simulink model "NEST"  (R2019a)
settings: Solver=VariableStepAuto  StartTime=0.0  StopTime=Inf  RelTol=1e-3
settings Model: Creator=marco  LastModifiedBy=luca
settings DataIOCC: ReturnWorkspaceOutputs=off
settings DebuggingCC: ArithmeticOperatorsInVariantConditions=warning

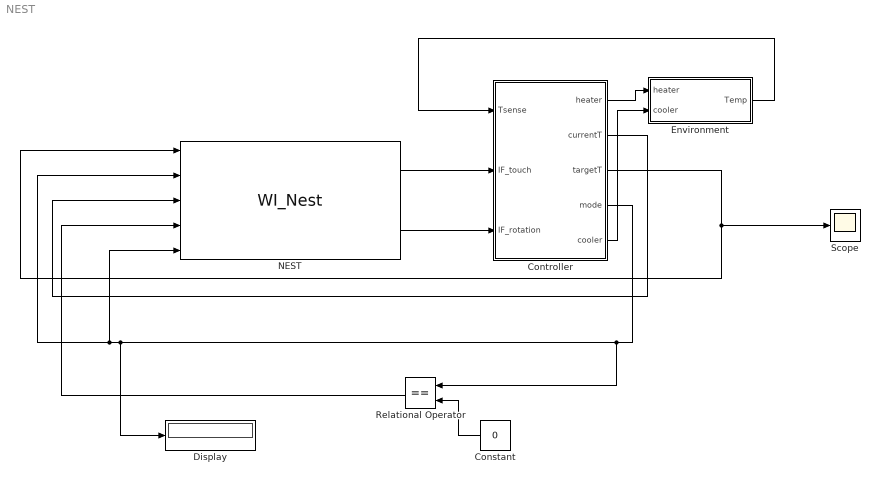
== system NEST ==
  Constant : Constant  Value=0  OutDataTypeStr=uint8
  Controller : Subsystem
  Display : Display
  Environment : Subsystem
  NEST : M-S-Function  FunctionName=WI_Nest
      mask Display:
      | port_label('output', 1, 'touch_lcd')
      | port_label('output', 2, 'rotational')
      | port_label('input', 1, 'centraltxt')
      | port_label('input', 2, 'statustxt')
      | port_label('input', 3, 'uppertxt')
      | port_label('input', 4, 'icon')
      | port_label('input', 5, 'mode')
  Relational Operator : RelationalOperator  Operator===  OutDataTypeStr=boolean  RndMeth=Simplest
  Scope : Scope
  wires:
  Controller/1(heater) -> Environment/1(heater)
  Environment/1(Temp) -> Controller/1(Tsense)
  NEST/1 -> Controller/2(IF_touch)
  NEST/2 -> Controller/3(IF_rotation)
  Controller/2(currentT) -> NEST/3
  Controller/3(targetT) -> Scope/1, NEST/1
  Controller/4(mode) -> Relational Operator/1, Display/1, NEST/5, NEST/2
  Relational Operator/1 -> NEST/4
  Constant/1 -> Relational Operator/2
  Controller/5("cooler ") -> Environment/2("cooler ")

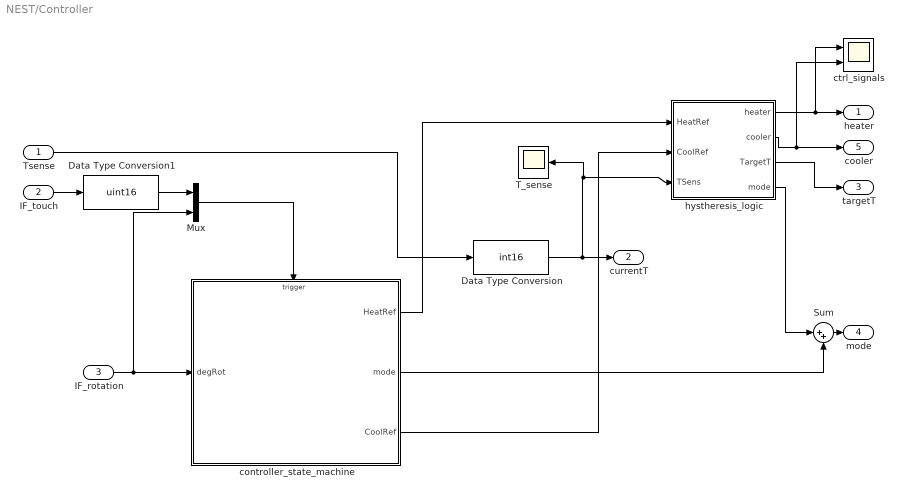
== system NEST/Controller ==
  Tsense : Inport
  IF_touch : Inport  Port=2
  IF_rotation : Inport  Port=3
  Data Type Conversion : DataTypeConversion  OutDataTypeStr=int16
  Data Type Conversion1 : DataTypeConversion  OutDataTypeStr=uint16
  Mux : Mux  Inputs=2
  Sum : Sum  Inputs=|++
  T_sense : Scope
  controller_state_machine : Stateflow chart  TreatAsAtomicUnit=on
  ctrl_signals : Scope  NumInputPorts=2
  hystheresis_logic : Stateflow chart  BlockKeywords=__PRM__SERIALIZED__DATA__:Stateflow Chart,Stateflow Diagram  TreatAsAtomicUnit=on
  heater : Outport
  currentT : Outport  Port=2  OutDataTypeStr=int16
  targetT : Outport  Port=3  OutDataTypeStr=int16
  mode : Outport  Port=4
  "cooler " : Outport  Port=5
  wires:
  hystheresis_logic/1(heater) -> ctrl_signals/1, heater/1
  Tsense/1 -> Data Type Conversion/1
  controller_state_machine/1(HeatRef) -> hystheresis_logic/1(HeatRef)
  controller_state_machine/2(mode) -> Sum/2
  IF_rotation/1 -> Mux/2, controller_state_machine/1(degRot)
  Mux/1 -> controller_state_machine/Trigger
  IF_touch/1 -> Data Type Conversion1/1
  Data Type Conversion/1 -> T_sense/1, hystheresis_logic/3(TSens), currentT/1
  Data Type Conversion1/1 -> Mux/1
  hystheresis_logic/2(cooler) -> ctrl_signals/2, "cooler "/1
  Sum/1 -> mode/1
  hystheresis_logic/4(mode) -> Sum/1
  controller_state_machine/3(CoolRef) -> hystheresis_logic/2(CoolRef)
  hystheresis_logic/3(TargetT) -> targetT/1

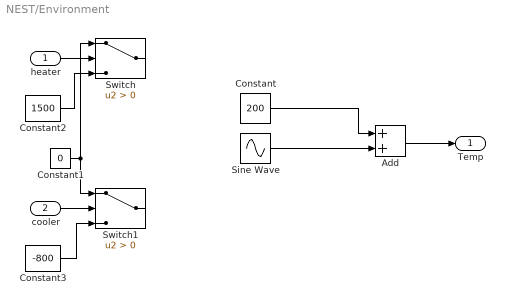
== system NEST/Environment ==
  heater : Inport
  "cooler " : Inport  Port=2
  Add : Sum
  Constant : Constant  Value=200
  Constant1 : Constant  Value=0
  Constant2 : Constant  Value=1500
  Constant3 : Constant  Value=-800
  Sine Wave : Sin  Amplitude=100  Frequency=0.001  SampleTime=0
  Switch : Switch  Criteria=u2 > Threshold
  Switch1 : Switch  Criteria=u2 > Threshold
  Temp : Outport
  wires:
  Add/1 -> Temp/1
  Sine Wave/1 -> Add/2
  Constant/1 -> Add/1
  heater/1 -> Switch/2
  "cooler "/1 -> Switch1/2
  Constant1/1 -> Switch/1, Switch1/1
  Constant2/1 -> Switch/3
  Constant3/1 -> Switch1/3

== stateflow chart NEST/Controller/hystheresis_logic ==
  state Heating
    en:heater=1;mode=2;TargetT=HeatRef
    ex:heater=0
  state Cooling
    en:cooler=1;mode=1;TargetT=CoolRef
    ex:cooler=0
  state Inactive
    en:mode=0
  note: se parto già con la temperatura alta o bassa devo valutare le transizioni mentre entro nella flowchart
  Heating -> Inactive : [TSens>HeatRef+5]
  Cooling -> Inactive : [TSens<CoolRef-5]
  Inactive -> Heating [order 1] : [TSens<HeatRef-5]
  Inactive -> Cooling [order 2] : [TSens>CoolRef+5]
  (default) -> Inactive : /{heater=0, cooler=0, mode=0, TargetT=TSens}
  data: heater output; cooler output; TargetT output int16; HeatRef input int16; CoolRef input int16; TSens input int16; mode output uint8

== stateflow chart NEST/Controller/controller_state_machine ==
  settings: executeAtInitialization=1
  state Off
    en: mode=100
  state On
    state ModeSetup
      en:mode=40
    state WeatherForecast
      en:mode=30
    state HeatingCooling
      en: mode=0
    state HeatingSetup
      en:mode=10
    state CoolingSetup
      en:mode=20
    (default) -> ModeSetup
    WeatherForecast -> ModeSetup : LCDButton
    CoolingSetup -> WeatherForecast : LCDButton
    ModeSetup -> HeatingCooling : LCDButton
    HeatingCooling -> HeatingSetup : LCDButton
    HeatingSetup -> CoolingSetup : LCDButton
  (default) -> Off : /{HeatRef=200; CoolRef=260; mode=0}
  Off -> On : LCDButton
  data: degRot input uint16; HeatRef output int16; mode output uint8; CoolRef output int16
  events: LCDButton input RISING_EDGE_EVENT; Changerot input EITHER_EDGE_EVENT
